simulink model "thermal_closed_loop_model"  (R2023a)
settings: Solver=ode23t  StartTime=0.0  StopTime=600  RelTol=1e-3
PostLoadFcn:
  | run('thermal_model_parameters.m')
  | run('thermal_harness_parameters.m')
  | run('thermal_variants_config.m')
values from neighbouring files (symbols this model uses):
  air_cp = 1004    [cathode_subsystem_parameters.m]    (also in thermal_subsystem_parameters.m)
  air_HC_min = 10    [cathode_subsystem_parameters.m]    (also in thermal_subsystem_parameters.m)
  air_HC_nom = 100    [cathode_subsystem_parameters.m]    (also in thermal_subsystem_parameters.m)
  air_rho = 1.2    [cathode_subsystem_parameters.m]    (also in thermal_subsystem_parameters.m)
  air_vel_nom = 1    [cathode_subsystem_parameters.m]    (also in thermal_subsystem_parameters.m)
  coolant_initial_pressure = 0.111325    [cathode_subsystem_parameters.m]    (also in thermal_subsystem_parameters.m)
  coolant_initial_temperature = 293.15    [cathode_subsystem_parameters.m]    (also in thermal_subsystem_parameters.m)
  coolant_tube_D = 0.05    [cathode_subsystem_parameters.m]    (also in thermal_subsystem_parameters.m)
  Hydrowell_VTS =     [Hydrowell_values_VLV.mat]
  radiator_area_air = 0.10260000000000001    (= 0.1026)    [cathode_subsystem_parameters.m]    (also in thermal_subsystem_parameters.m)
  radiator_area_fins = 2.5436250000000005    (= 2.543625)    [cathode_subsystem_parameters.m]    (also in thermal_subsystem_parameters.m)
  radiator_area_primary = 0.44452500000000011    (= 0.444525)    [cathode_subsystem_parameters.m]    (also in thermal_subsystem_parameters.m = 2 * radiator_tube_length * radiator_width * (radiator_fin_ro)
  radiator_n_tubes = 20    [cathode_subsystem_parameters.m]    (also in thermal_subsystem_parameters.m)
  radiator_tube_height = 0.0015    [cathode_subsystem_parameters.m]    (also in thermal_subsystem_parameters.m)
  radiator_tube_length = 0.45    [cathode_subsystem_parameters.m]    (also in thermal_subsystem_parameters.m)
  radiator_width = 0.025    [cathode_subsystem_parameters.m]    (also in thermal_subsystem_parameters.m)
  tcp_time_constant = 2    [cathode_subsystem_parameters.m]    (also in thermal_subsystem_parameters.m)
undefined symbols (not defined in the file or in its folder): sigbuilder_block, stack
libraries: fl_lib x153, nesl_utility x122, SimscapeFluids_lib x16, slpidlib x5, simulink x1
(part 1 of 8)
settings Model: Creator=adrian.taveras  LastModifiedBy=adrian.taveras
settings SolverCC: MaxConsecutiveMinStep=10
settings OptimizationCC: ReuseModelBlockBuffer=off
settings SimscapeCC: SimscapeLogType=all

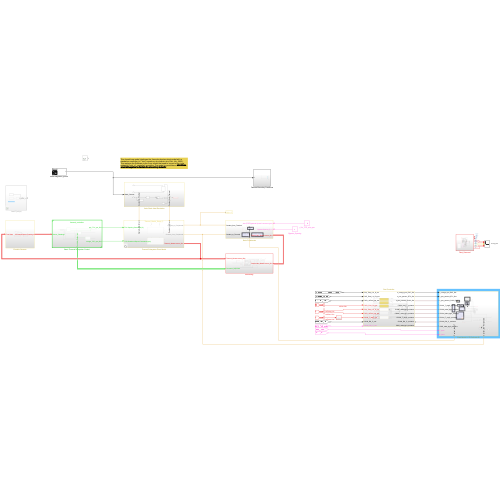
[thumbnail: Simulink's stored preview of the top-level diagram]
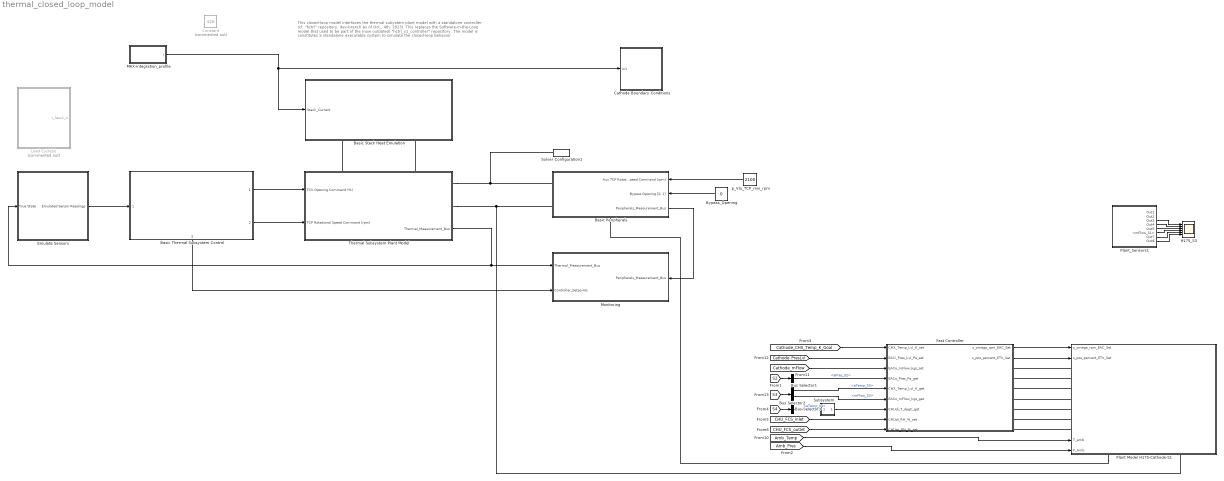
== system thermal_closed_loop_model ==
  note: This closed-loop model interfaces the thermal subystem plant model with a standalone controller (cf. "hctrl" repository, dev-branch as of Oct., 4th, 2023).
      | This replaces the Software-in-the-Loop model that used to be part of the (now outdated) "hctrl_v1_controller" repository. The model is constitutes a standalone executable system to simulate the closed-loop behavior .
  Basic Peripherals : Subsystem
      settings: PortSchema="{\"entries\":[{\"content\":{\"sides\":[{\"content\":{\"connectorIds\":[\"LConn1\",\"LConn2\"]},\"type\":\"ConnectorPlacement.EquallySpacedRectSide\",\"uuid\":\"3fb1bffc-06de-43a0-ba54-014616fc6cc1\"},{\"content\":{\"connectorIds\":[\"In1\",\"In2\",\"Out1\"],\"side\":\"RIGHT\"},\"type\":\"ConnectorPlacement.EquallySpacedRectSide\",\"uuid\":\"58405954-0a26-4c47-92cd-2c539f5c2dc2\"},{\"content\":{\"side\":\"TOP\"},\"type\":\"ConnectorPlacement.EquallySpacedRectSide\",\"uuid\":\"fb935e14-bdb8-42f8-ab88-5e819e25323e\"},{\"content\":{\"connectorIds\":[\"RConn1\"],\"side\":\"BOTTOM\"},\"type\":\"ConnectorPlacement.EquallySpacedRectSide\",\"uuid\":\"4a5f4864-27a3-41f8-b148-25be1e393b46\"}]},\"type\":\"ConnectorPlacement.EquallySpacedConnector\",\"uuid\":\"bd863423-caf1-4028-a014-0e522635d1ca\"}],\"packageUris\":[\"http://schema.mathworks.com/mf0/Connector/R2020b\"],\"version\":\"1.0\"}"
  Basic Stack Heat Emulation : Subsystem
      settings: PortSchema="{\"entries\":[{\"content\":{\"sides\":[{\"content\":{\"connectorIds\":[\"In1\"]},\"type\":\"ConnectorPlacement.EquallySpacedRectSide\",\"uuid\":\"3fb1bffc-06de-43a0-ba54-014616fc6cc1\"},{\"content\":{\"side\":\"RIGHT\"},\"type\":\"ConnectorPlacement.EquallySpacedRectSide\",\"uuid\":\"58405954-0a26-4c47-92cd-2c539f5c2dc2\"},{\"content\":{\"side\":\"TOP\"},\"type\":\"ConnectorPlacement.EquallySpacedRectSide\",\"uuid\":\"fb935e14-bdb8-42f8-ab88-5e819e25323e\"},{\"content\":{\"connectorIds\":[\"RConn1\",\"RConn2\"],\"side\":\"BOTTOM\"},\"type\":\"ConnectorPlacement.EquallySpacedRectSide\",\"uuid\":\"52bc4db1-df79-4132-9e52-2843fbef2d40\"}]},\"type\":\"ConnectorPlacement.EquallySpacedConnector\",\"uuid\":\"bd863423-caf1-4028-a014-0e522635d1ca\"}],\"packageUris\":[\"http://schema.mathworks.com/mf0/Connector/R2020b\"],\"version\":\"1.0\"}"
  Basic Thermal Subsystem Control : Subsystem  TreatAsAtomicUnit=on  SystemSampleTime=0.05  ReferencedSubsystem=thermal_controller
      settings: RTWFcnNameOpts=Use subsystem name  RTWFileNameOpts=Use subsystem name  PortSchema="{\"entries\":[{\"content\":{\"sides\":[{\"content\":{\"connectorIds\":[\"In1\"]},\"type\":\"ConnectorPlacement.EquallySpacedRectSide\",\"uuid\":\"5ce399fd-075d-47cf-80d1-ee07a0b07c67\"},{\"content\":{\"connectorIds\":[\"Out1\",\"Out2\"],\"side\":\"RIGHT\"},\"type\":\"ConnectorPlacement.EquallySpacedRectSide\",\"uuid\":\"2f333d4b-83ed-4fad-b30d-41906106278f\"},{\"content\":{\"side\":\"TOP\"},\"type\":\"ConnectorPlacement.EquallySpacedRectSide\",\"uuid\":\"ce20a072-8b2c-48f8-86cd-e043d93c9dd9\"},{\"content\":{\"connectorIds\":[\"Out3\"],\"side\":\"BOTTOM\"},\"type\":\"ConnectorPlacement.EquallySpacedRectSide\",\"uuid\":\"72f45d63-3937-4d85-84da-630e4ae9e6af\"}]},\"type\":\"ConnectorPlacement.EquallySpacedConnector\",\"uuid\":\"e1990042-c5e7-41f2-bf10-f2665fc49181\"}],\"packageUris\":[\"http://schema.mathworks.com/mf0/Connector/R2020b\"],\"version\":\"1.0\"}"
  Bus Selector1 : BusSelector  OutputSignals=aPres_S2
  Bus Selector2 : BusSelector  OutputSignals=aTemp_S3,mFlow_S3
  Bus Selector3 : BusSelector  OutputSignals=aTemp_S4
  Bypass_Opening : Constant  Value=0
  Cathode Boundary Conditions : Subsystem
  Constant : Constant  Commented=on  Value=426
  Emulate Sensors : Subsystem
  Fast Controller : Subsystem
      settings: PortSchema="{\"entries\":[{\"content\":{\"sides\":[{\"content\":{\"connectorIds\":[\"Out1\",\"Out2\",\"LConn1\",\"LConn2\",\"LConn3\",\"LConn4\",\"LConn5\",\"LConn6\",\"LConn7\"]},\"type\":\"ConnectorPlacement.EquallySpacedRectSide\",\"uuid\":\"fec6d33c-3ad3-4174-acdc-3a3b9e5715f4\"},{\"content\":{\"connectorIds\":[\"In1\",\"In2\",\"In3\",\"In4\",\"In5\",\"In6\",\"In7\",\"In8\",\"In9\"],\"side\":\"RIGHT\"},\"type\":\"ConnectorPlacement.EquallySpacedRectSide\",\"uuid\":\"4aee90de-c0ab-447d-83f7-53a254285efe\"},{\"content\":{\"side\":\"TOP\"},\"type\":\"ConnectorPlacement.EquallySpacedRectSide\",\"uuid\":\"94b2adb1-5e3a-4413-84ea-fe1e13b8a59d\"}]},\"type\":\"ConnectorPlacement.EquallySpacedConnector\",\"uuid\":\"aca8449a-2e64-4d0b-80a0-10fe30b1ea20\"}],\"packageUris\":[\"http://schema.mathworks.com/mf0/Connector/R2020b\"],\"version\":\"1.0\"}"
  H175_S3 : Scope  NumInputPorts=6
  Load Cycle(s) : Subsystem  Commented=on
  MAX-integration_profile : Subsystem  Tag=STV Subsys  LoadFcn=sigbuilder_block('load');  StartFcn=sigbuilder_block('start');  StopFcn=sigbuilder_block('stop');  ClipboardFcn=sigbuilder_block('clipboard');  mask(Sigbuilder block){tuvar=[0:10]}
      mask help: Simulink:masks:SigbuilderBlock_MD
      mask init:
      | if ~strcmp(get_param(bdroot(gcbh),'SimulationStatus'),'stopped') tuvar = sigbuilder_block('maskInit'); end
      settings: CopyFcn=sigbuilder_block('copy');  DeleteFcn=sigbuilder_block('delete');  ModelCloseFcn=sigbuilder_block('modelClose');  PreSaveFcn=sigbuilder_block('preSave');  PauseFcn=sigbuilder_block('pause');  ContinueFcn=sigbuilder_block('continue');  NameChangeFcn=sigbuilder_block('namechange');  OpenFcn=sigbuilder_block('open',[6 30.75 1428 715.5 ]);  CloseFcn=sigbuilder_block('close');
      mask Display: plot(0, 0, 100, 100,[2, 2, 32, 32, 2], [68, 8, 8, 68, 68],[32, 2], [38, 38], [32, 19, 2],[53, 60, 44], [32, 17, 17, 2],[16, 16, 31, 31]);txt = getActiveGroup(gcbh);text(2, 100, txt,'verticalAlignment', 'top');
  Monitoring : Subsystem
      settings: PortSchema="{\"entries\":[{\"content\":{\"sides\":[{\"content\":{\"connectorIds\":[\"In1\",\"In2\"]},\"type\":\"ConnectorPlacement.EquallySpacedRectSide\",\"uuid\":\"c7cb1208-b668-4b39-b890-dd3e20c5f08d\"},{\"content\":{\"connectorIds\":[\"In3\"],\"side\":\"RIGHT\"},\"type\":\"ConnectorPlacement.EquallySpacedRectSide\",\"uuid\":\"340204d2-358d-42ec-bbb6-f536bf598eab\"},{\"content\":{\"side\":\"TOP\"},\"type\":\"ConnectorPlacement.EquallySpacedRectSide\",\"uuid\":\"3db79fdc-6863-4ab5-88bc-fd1ec2b642bb\"}]},\"type\":\"ConnectorPlacement.EquallySpacedConnector\",\"uuid\":\"cd44049f-98c6-404f-bd6e-056e1be05d3b\"}],\"packageUris\":[\"http://schema.mathworks.com/mf0/Connector/R2020b\"],\"version\":\"1.0\"}"
  Plant Model H175-Cathode-S1 : Subsystem
      settings: PortSchema="{\"entries\":[{\"content\":{\"sides\":[{\"content\":{\"connectorIds\":[\"In1\",\"In2\",\"LConn1\",\"LConn2\",\"LConn3\",\"LConn4\",\"LConn5\",\"LConn6\",\"LConn7\",\"In3\",\"In4\"]},\"type\":\"ConnectorPlacement.EquallySpacedRectSide\",\"uuid\":\"e3b30cb5-20d3-4977-927f-9fea068a9234\"},{\"content\":{\"side\":\"RIGHT\"},\"type\":\"ConnectorPlacement.EquallySpacedRectSide\",\"uuid\":\"2d547627-9665-492a-afa4-fcc16b1173a1\"},{\"content\":{\"side\":\"TOP\"},\"type\":\"ConnectorPlacement.EquallySpacedRectSide\",\"uuid\":\"4ee6a80a-af1f-40b1-aa59-916ec7fe1294\"},{\"content\":{\"connectorIds\":[\"RConn1\",\"RConn2\"],\"side\":\"BOTTOM\"},\"type\":\"ConnectorPlacement.EquallySpacedRectSide\",\"uuid\":\"f96b90ea-bf7b-40d9-b9ad-d818d5da9577\"}]},\"type\":\"ConnectorPlacement.EquallySpacedConnector\",\"uuid\":\"0d82e4d1-cc18-4647-90fc-0df577891cdc\"}],\"packageUris\":[\"http://schema.mathworks.com/mf0/Connector/R2020b\"],\"version\":\"1.0\"}"
  Plant_Sensors1 : Subsystem
  Solver Configuration1 : nesl_utility/Solver Configuration  PhysicalDomain=network_engine_domain  SubClassName=solver  LeftPortType=input  RightPortType=generic  Tones=[]  Harmonics=[]  SimulateNoise=off  Profile=off  UseLocalSampling=off  EnableSwitchedLinearOptims=on  FrequencyDomain=off  UseCCode=off  RelTol=0.001  AbsTol=1e-06  MinStep=1e-09  ToWorkspace=off  RevertToSquareIcSolve=off  NumHomotopyIterations=100  PhasorMode=off  PhasorModeNumHarmonics=1  ConsistencySolver=NEWTON_XTOL_AFTER_FTOL  IndexReductionMethod=DerivativeReplacement  DoDC=on  ResidualTolerance=1e-09  ConsistencyTolSource=GLOBAL  ConsistencyAbsTol=0.001  ConsistencyRelTol=0.001  ConsistencyTolFactor=0.001  UseLocalSolver=on  LocalSolverChoice=NE_BACKWARD_EULER_ADVANCER  ResolveIndetEquations=on  FunctionEvalNumThread=1  LocalSolverSampleTime=0.001  DoFixedCost=on  MaxNonlinIter=3  MaxModeIter=2  ComputeImpulses=off  ImpulseIterations=2  LinearAlgebra=auto  LinearAlgebraNumThread=0  EquationFormulation=NE_TIME_EF  DelaysMemoryBudget=1024  AutomaticFiltering=off  FilteringTimeConstant=0.001  PartitionStorageMethod=AS_NEEDED  PartitionMemoryBudget=1024  PartitionMethod=ROBUST
  Subsystem : Subsystem
  Thermal Subsystem Plant Model : Subsystem  Variant=on
      settings: PortSchema="{\"entries\":[{\"content\":{\"sides\":[{\"content\":{\"connectorIds\":[\"In1\",\"In2\"]},\"type\":\"ConnectorPlacement.EquallySpacedRectSide\",\"uuid\":\"c406812b-8c92-4602-a172-62ad771a81a9\"},{\"content\":{\"connectorIds\":[\"RConn1\",\"RConn2\",\"Out1\"],\"side\":\"RIGHT\"},\"type\":\"ConnectorPlacement.EquallySpacedRectSide\",\"uuid\":\"78b6fff5-4256-4005-adaa-354cc2ed5b7d\"},{\"content\":{\"connectorIds\":[\"LConn1\",\"LConn2\"],\"side\":\"TOP\"},\"type\":\"ConnectorPlacement.EquallySpacedRectSide\",\"uuid\":\"1d5f4f72-4393-4f38-b9ce-f5bde53d6a3a\"}]},\"type\":\"ConnectorPlacement.EquallySpacedConnector\",\"uuid\":\"f62a8404-8485-4e42-883e-e8d18b630e2d\"}],\"packageUris\":[\"http://schema.mathworks.com/mf0/Connector/R2020b\"],\"version\":\"1.0\"}"
  p_Vlo_TCP_min_rpm : Constant  Value=2100
  wires:
  Thermal Subsystem Plant Model/1(Thermal_Measurement_Bus) -> Emulate Sensors/1(True State), Monitoring/1(Thermal_Measurement_Bus)
  Emulate Sensors/1(Emulated Sensor Readings) -> Basic Thermal Subsystem Control/1
  p_Vlo_TCP_min_rpm/1 -> Basic Peripherals/1(Aux TCP Rotational Speed Command (rpm))
  Basic Peripherals/1(Peripherals_Measurement_Bus) -> Monitoring/3(Peripherals_Measurement_Bus)
  Basic Thermal Subsystem Control/3 -> Monitoring/2(Controller_Setpoints)
  Bypass_Opening/1 -> Basic Peripherals/2("Bypass Opening [0, 1]")
  Basic Thermal Subsystem Control/1 -> Thermal Subsystem Plant Model/1(TCV Opening Command (%))
  Basic Thermal Subsystem Control/2 -> Thermal Subsystem Plant Model/2(TCP Rotational Speed Command (rpm))
  [Amb_Temp] -> Plant Model H175-Cathode-S1/3(T_amb)
  Bus Selector1/1 -> Fast Controller/4(EACo_Pres_Pa_get)  "<aPres_S2>"
  Bus Selector3/1 -> Subsystem/1(<aTemp_S4>)  "<aTemp_S4>"
  Bus Selector2/1 -> Fast Controller/5(CHX_Temp_Lvl_K_get)  "<aTemp_S3>"
  [S3] -> Bus Selector2/1
  [Cathode_CHX_Temp_K_Goal] -> Fast Controller/1(CHX_Temp_Lvl_K_set)
  Fast Controller/2(s_pos_percent_ETV_Set) -> Plant Model H175-Cathode-S1/2(s_pos_percent_ETV_Set)
  Fast Controller/1(s_omega_rpm_EAC_Set) -> Plant Model H175-Cathode-S1/1(s_omega_rpm_EAC_Set)
  [CHU_FCS_outlet] -> Fast Controller/9(CHUwi_RH_%_set)
  Bus Selector2/2 -> Fast Controller/6(EACo_mFlow_kgs_get)  "<mFlow_S3>"
  Subsystem/1(Out1) -> Fast Controller/7(CHUdi_T_degC_get)
  [S4] -> Bus Selector3/1
  Plant_Sensors1/7(Out7) -> H175_S3/5
  [Cathode_PresLvl] -> Fast Controller/2(EACi_Pres_Lvl_Pa_set)
  [CHU_FCS_inlet] -> Fast Controller/8(CHUdi_RH_%_set)
  Plant_Sensors1/5(Out5) -> H175_S3/3
  Plant_Sensors1/4(Out4) -> H175_S3/2
  Plant_Sensors1/3(Out3) -> H175_S3/1
  Plant_Sensors1/8(Out8) -> H175_S3/6
  [Cathode_mFlow] -> Fast Controller/3(EACo_mFlow_kgs_set)
  [S2] -> Bus Selector1/1
  MAX-integration_profile/1(I) -> Basic Stack Heat Emulation/1(Stack_Current), Cathode Boundary Conditions/1(In1)
  Plant_Sensors1/6(<mFlow_S1>) -> H175_S3/4
  [Amb_Pres] -> Plant Model H175-Cathode-S1/4(P_Amb)
  connections:
  Thermal Subsystem Plant Model/LConn2 -- Basic Stack Heat Emulation/RConn2
  Thermal Subsystem Plant Model/LConn1 -- Basic Stack Heat Emulation/RConn1
  Solver Configuration1/RConn1 -- Thermal Subsystem Plant Model/RConn1 -- Basic Peripherals/LConn1
  Thermal Subsystem Plant Model/RConn2 -- Plant Model H175-Cathode-S1/RConn2 -- Basic Peripherals/LConn2
  Plant Model H175-Cathode-S1/LConn6 -- Fast Controller/LConn6
  Plant Model H175-Cathode-S1/LConn7 -- Fast Controller/LConn7
  Plant Model H175-Cathode-S1/LConn4 -- Fast Controller/LConn4
  Plant Model H175-Cathode-S1/LConn5 -- Fast Controller/LConn5
  Plant Model H175-Cathode-S1/LConn2 -- Fast Controller/LConn2
  Plant Model H175-Cathode-S1/LConn3 -- Fast Controller/LConn3
  Plant Model H175-Cathode-S1/LConn1 -- Fast Controller/LConn1
  Plant Model H175-Cathode-S1/RConn1 -- Basic Peripherals/RConn1

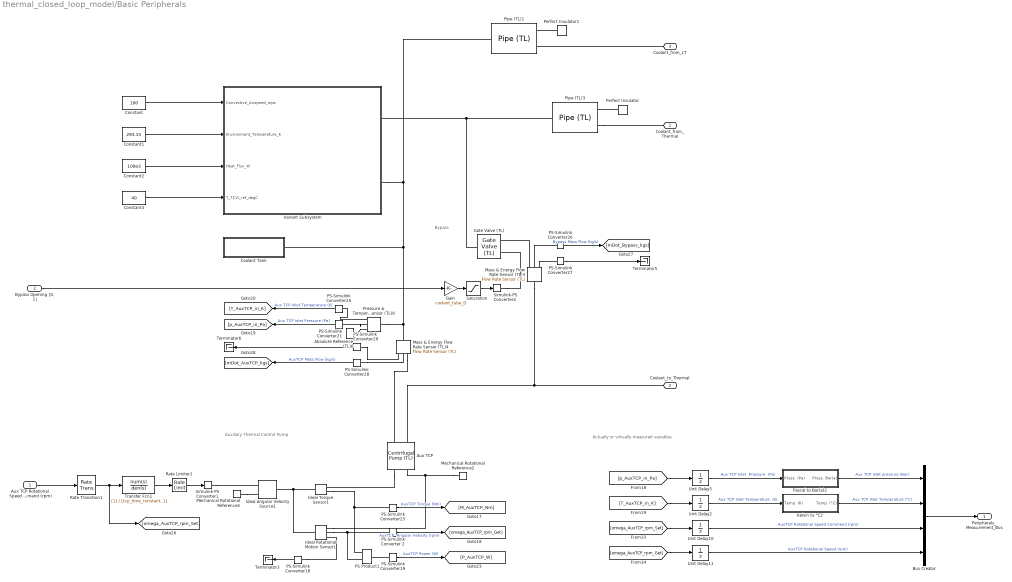
== system thermal_closed_loop_model/Basic Peripherals ==
  note: Auxiliary Thermal Control Pump
  note: Actually or virtually measured variables
  note: Bypass
  Aux TCP Rotational Speed Command (rpm) : Inport
  "Bypass Opening [0, 1]" : Inport  Port=2
  Absolute Reference (TL)6 : fl_lib/Thermal Liquid/Elements/Absolute Reference (TL)
  Aux TCP : SimscapeFluids_lib/Thermal Liquid/Pumps & Motors/Centrifugal Pump (TL)  pump_parameterization=fluids.thermal_liquid.pumps_motors.enum.CentrifugalPumpParameterization.Nominal  capacity_ref_nominal=6000/60 lpm  head_ref_nominal=|  power_ref_nominal=0.3 kW  head_ref_max=|  capacity_ref_max=12000/60 lpm  omega_ref_analytic=3500 rpm  flow_rate_1D_TLU=[1000, 2000, 3000, 4000, 5000, 6000, 7000, 8000, 9000, 1000] lpm  head_1D_TLU=[50, 47.5, 45, 40, 35, 25] m  power_1D_TLU=[.6, .75, .85, .93, .98, .99] kW  omega_ref_1D=3500 rpm  rho_ref_1D=998.21 kg/m^3  omega_threshold_factor=1e-2  flow_rate_2D_TLU=[16.67, 23.33, 30, 40, 53.33, 60] lpm  omega_2D_TLU=[2450, 2800, 3150, 3500] rpm  head_2D_TLU=[25, 32.7, 42.5, 50; 24, 31.7, 41, 49; 22.7, 30.5, 39, 47.5; 20, 28, 36, 45; 15.7, 24, 32, 40; 12.5, 21, 29.5, 37.5] m  power_2D_TLU=[.28, .38, .5, .6; .31, .41, .55, .68; .33, .44, .6, .75; .36, .48, .65, .83; .38, .53, .72, .93; .39, .55, .75, .97] kW  rho_ref_2D=998.21 kg/m^3  diameter_ratio=1  mech_orientation=fluids.thermal_liquid.pumps_motors.enum.CentrifugalPumpMechOrientation.Positive  area=9.6211275016187417927918453612935e-4 m^2
      head_ref_nominal=|
      | 1.2*10^5/(1000*9.81)
      |  m
      head_ref_max=|
      | 1.55*10^5/(1000*9.81)
      |  m
      settings: InternalSimscapePortConfiguration="{\"Bottom\":[],\"Left\":[{\"id\":\"A\",\"label\":\"A\",\"type\":\"foundation.thermal_liquid.thermal_liquid\"},{\"id\":\"B\",\"label\":\"B\",\"type\":\"foundation.thermal_liquid.thermal_liquid\"}],\"Right\":[{\"id\":\"R\",\"label\":\"R\",\"type\":\"foundation.mechanical.rotational.rotational\"},{\"id\":\"C\",\"label\":\"C\",\"type\":\"foundation.mechanical.rotational.rotational\"}],\"Top\":[]}"
  Bus Creator : BusCreator  Inputs=4
  Constant : Constant  Value=100
  Constant1 : Constant  Value=293.15
  Constant2 : Constant  Value=100e3
  Constant3 : Constant  Value=40
  Coolant Tank : Subsystem  Tag=PublishSubsystem  mask(Coolant Tank){A=1, x_init=0.08}
      mask prompts: A "Tank area (m^2)"; x_init "Initial coolant level (m)"
      mask help: This subsystem models an expansion tank for the coolant system.
  Gain : Gain  Gain=coolant_tube_D
  Gate Valve (TL) : SimscapeFluids_lib/Thermal Liquid/Valves & Orifices/Flow Control Valves/Gate Valve (TL)  diam_orifice=coolant_tube_D*0.9 m  S_min=0 m  area_leak=1e-12 m^2  smoothing_factor=0.01  area=pi*coolant_tube_D^2/4 m^2  Cd=0.7  Re_c=12
      settings: InternalSimscapePortConfiguration="{\"Bottom\":[],\"Left\":[{\"id\":\"A\",\"label\":\"A\",\"type\":\"foundation.thermal_liquid.thermal_liquid\"},{\"id\":\"S\",\"label\":\"S\",\"type\":\"input\"}],\"Right\":[{\"id\":\"B\",\"label\":\"B\",\"type\":\"foundation.thermal_liquid.thermal_liquid\"}],\"Top\":[]}"
  Ideal Angular Velocity Source1 : fl_lib/Mechanical/Mechanical Sources/Ideal Angular Velocity Source
  Ideal Rotational Motion Sensor1 : fl_lib/Mechanical/Mechanical Sensors/Ideal Rotational Motion Sensor  reference=foundation.enum.MeasurementReference.difference  acceleration_port=false  velocity_port=true  position_port=true  wrap_angle=false  offset=0 rad
  Ideal Torque Sensor1 : fl_lib/Mechanical/Mechanical Sensors/Ideal Torque Sensor
  Kelvin to °C2 : Subsystem
  Mass & Energy Flow Rate Sensor (TL)3 : fl_lib/Thermal Liquid/Sensors/Flow Rate Sensor (TL)  mass_flow_measure=true  volumetric_flow_measure=false  energy_flow_measure=true
      settings: InternalSimscapePortConfiguration="{\"Bottom\":[{\"id\":\"PHI\",\"label\":\"φ\",\"type\":\"output\"}],\"Left\":[{\"id\":\"A\",\"label\":\"A\",\"type\":\"foundation.thermal_liquid.thermal_liquid\"}],\"Right\":[{\"id\":\"B\",\"label\":\"B\",\"type\":\"foundation.thermal_liquid.thermal_liquid\"},{\"id\":\"M\",\"label\":\"M\",\"type\":\"output\"}],\"Top\":[]}"
  Mass & Energy Flow Rate Sensor (TL)4 : fl_lib/Thermal Liquid/Sensors/Flow Rate Sensor (TL)  mass_flow_measure=true  volumetric_flow_measure=false  energy_flow_measure=true
      settings: InternalSimscapePortConfiguration="{\"Bottom\":[{\"id\":\"PHI\",\"label\":\"φ\",\"type\":\"output\"}],\"Left\":[{\"id\":\"A\",\"label\":\"A\",\"type\":\"foundation.thermal_liquid.thermal_liquid\"}],\"Right\":[{\"id\":\"B\",\"label\":\"B\",\"type\":\"foundation.thermal_liquid.thermal_liquid\"},{\"id\":\"M\",\"label\":\"M\",\"type\":\"output\"}],\"Top\":[]}"
  Mechanical Rotational Reference2 : fl_lib/Mechanical/Rotational Elements/Mechanical Rotational Reference
  Mechanical Rotational Reference4 : fl_lib/Mechanical/Rotational Elements/Mechanical Rotational Reference
  PS Product1 : fl_lib/Physical Signals/Functions/PS Product
  PS-Simulink Converter 2 : nesl_utility/PS-Simulink Converter  PhysicalDomain=network_engine_domain  SubClassName=ps_output  LeftPortType=input  RightPortType=output  PseudoPeriodic=off  Frequencies=[]  VectorFormat=1-D array  Unit=rpm  AffineConversion=off
  PS-Simulink Converter{18,20..21,26..29} (7 alike) : nesl_utility/PS-Simulink Converter  PhysicalDomain=network_engine_domain  SubClassName=ps_output  LeftPortType=input  RightPortType=output  PseudoPeriodic=off  Frequencies=[]  VectorFormat=inherit  Unit=inherit  AffineConversion=off
  PS-Simulink Converter19 : nesl_utility/PS-Simulink Converter  PhysicalDomain=network_engine_domain  SubClassName=ps_output  LeftPortType=input  RightPortType=output  PseudoPeriodic=off  Frequencies=[]  VectorFormat=inherit  Unit=W  AffineConversion=off
  PS-Simulink Converter25 : nesl_utility/PS-Simulink Converter  PhysicalDomain=network_engine_domain  SubClassName=ps_output  LeftPortType=input  RightPortType=output  PseudoPeriodic=off  Frequencies=[]  VectorFormat=inherit  Unit=N*m  AffineConversion=off
  Pascal to Bar(a)2 : Subsystem
  Perfect Insulator : fl_lib/Thermal/Thermal Elements/Perfect Insulator  T_specify=off  T_priority=None  T=293.15 K  T_nominal_specify=off  T_nominal_unit=K  T_nominal_value=1
  Perfect Insulator1 : fl_lib/Thermal/Thermal Elements/Perfect Insulator  T_specify=off  T_priority=None  T=293.15 K  T_nominal_specify=off  T_nominal_unit=K  T_nominal_value=1
  Pipe (TL)1 : fl_lib/Thermal Liquid/Elements/Pipe (TL)  length=1 m  area=pi*(coolant_tube_D/2)^2/4 m^2  Dh=pi*coolant_tube_D*.5*0.9 m  length_add=1 m  roughness=15e-6 m  Re_lam=2000  Re_tur=4000  shape_factor=64  Nu_lam=3.66  dynamic_compressibility=simscape.enum.onoff.on  inertia=simscape.enum.onoff.off  p0=coolant_initial_pressure MPa  T0=coolant_initial_temperature K  mdot0=0 kg/s
  Pipe (TL)3 : fl_lib/Thermal Liquid/Elements/Pipe (TL)  length=1 m  area=pi*coolant_tube_D^2/4 m^2  Dh=pi*coolant_tube_D*0.9 m  length_add=1 m  roughness=15e-6 m  Re_lam=2000  Re_tur=4000  shape_factor=64  Nu_lam=3.66  dynamic_compressibility=simscape.enum.onoff.on  inertia=simscape.enum.onoff.off  p0=coolant_initial_pressure MPa  T0=coolant_initial_temperature K  mdot0=0 kg/s
  Pressure & Temperature Sensor (TL)6 : fl_lib/Thermal Liquid/Sensors/Pressure & Temperature Sensor (TL)  reference=foundation.enum.MeasurementReference.difference  pressure=true  pressure_spec=foundation.enum.PressureMeasementSpec.Absolute  temperature=true
      settings: InternalSimscapePortConfiguration="{\"Bottom\":[{\"id\":\"T\",\"label\":\"T\",\"type\":\"output\"}],\"Left\":[{\"id\":\"A\",\"label\":\"A\",\"type\":\"foundation.thermal_liquid.thermal_liquid\"}],\"Right\":[{\"id\":\"B\",\"label\":\"B\",\"type\":\"foundation.thermal_liquid.thermal_liquid\"},{\"id\":\"P\",\"label\":\"P\",\"type\":\"output\"}],\"Top\":[]}"
  Rate Limiter1 : RateLimiter  RisingSlewLimit=1000  FallingSlewLimit=-1000  SampleTimeMode=inherited
  Rate Transition1 : RateTransition
  Saturation : Saturate  UpperLimit=coolant_tube_D  LowerLimit=0
  Simulink-PS Converter1 : nesl_utility/Simulink-PS Converter  PhysicalDomain=network_engine_domain  SubClassName=ps_input  LeftPortType=input  RightPortType=output  PseudoPeriodic=off  Frequencies=[]  NoiseDistribution=none  NoiseParameters=[]  Unit=rpm  AffineConversion=off  FilteringAndDerivatives=provide  SimscapeFilterOrder=1  InputFilterTimeConstant=0.001  UdotUserProvided=0
  Simulink-PS Converter4 : nesl_utility/Simulink-PS Converter  PhysicalDomain=network_engine_domain  SubClassName=ps_input  LeftPortType=input  RightPortType=output  PseudoPeriodic=off  Frequencies=[]  NoiseDistribution=none  NoiseParameters=[]  Unit=1  AffineConversion=off  FilteringAndDerivatives=provide  SimscapeFilterOrder=1  InputFilterTimeConstant=0.001  UdotUserProvided=0
  Terminator3 : Terminator
  Terminator5 : Terminator
  Terminator6 : Terminator
  Transfer Fcn1 : TransferFcn  Denominator=[tcp_time_constant, 1]  ContinuousStateAttributes='tcv_opening'
  Unit Delay10 : UnitDelay  SampleTime=-1  HasFrameUpgradeWarning=on
  Unit Delay11 : UnitDelay  SampleTime=-1  HasFrameUpgradeWarning=on
  Unit Delay2 : UnitDelay  InitialCondition=coolant_initial_temperature  SampleTime=-1  HasFrameUpgradeWarning=on
  Unit Delay5 : UnitDelay  InitialCondition=coolant_initial_pressure  SampleTime=-1  HasFrameUpgradeWarning=on
  Variant Subsystem : Subsystem  Variant=on
  Coolant_from_Thermal : PMIOPort  Side=Left
  Coolant_to_Thermal : PMIOPort  Port=2  Side=Left
  Coolant_from_LT : PMIOPort  Port=3  Side=Right
  Peripherals_Measurement_Bus : Outport
  wires:
  Aux TCP Rotational Speed Command (rpm)/1 -> Rate Transition1/1
  PS-Simulink Converter29/1 -> Terminator6/1
  PS-Simulink Converter20/1 -> [T_AuxTCP_in_K]  "Aux TCP Inlet Temperature (K)"
  PS-Simulink Converter21/1 -> [p_AuxTCP_in_Pa]  "Aux TCP Inlet Pressure (Pa)"
  PS-Simulink Converter19/1 -> [P_AuxTCP_W]  "AuxTCP Power (W)"
  Rate Transition1/1 -> [omega_AuxTCP_rpm_Set], Transfer Fcn1/1
  PS-Simulink Converter 2/1 -> [omega_AuxTCP_rpm_Get]  "AuxTCP  Angular Velocity (rpm)"
  PS-Simulink Converter25/1 -> [M_AuxTCP_Nm]  "AuxTCP Torque (Nm)"
  PS-Simulink Converter18/1 -> Terminator3/1
  Rate Limiter1/1 -> Simulink-PS Converter1/1
  Transfer Fcn1/1 -> Rate Limiter1/1
  PS-Simulink Converter28/1 -> [mDot_AuxTCP_kgs]  "AuxTCP Mass Flow (kg/s)"
  Pascal to Bar(a)2/1(Press. Bar(a)) -> Bus Creator/1  "Aux TCP Inlet pressure (Bar)"
  Unit Delay10/1 -> Bus Creator/3  "AuxTCP Rotational Speed Command (rpm)"
  Kelvin to °C2/1(Temp. (°C)) -> Bus Creator/2  "Aux TCP Inlet Temperature (°C)"
  [omega_AuxTCP_rpm_Get] -> Unit Delay11/1
  Unit Delay2/1 -> Kelvin to °C2/1(Temp. (K))  "Aux TCP Inlet Temperature  (K)"
  Unit Delay5/1 -> Pascal to Bar(a)2/1(Press. (Pa))  "Aux TCP Inlet  Pressure  (Pa)"
  Unit Delay11/1 -> Bus Creator/4  "AuxTCP Rotational Speed (rpm)"
  [p_AuxTCP_in_Pa] -> Unit Delay5/1
  [T_AuxTCP_in_K] -> Unit Delay2/1
  [omega_AuxTCP_rpm_Set] -> Unit Delay10/1
  Bus Creator/1 -> Peripherals_Measurement_Bus/1
  Constant/1 -> Variant Subsystem/1(Convective_Airspeed_mps)
  Constant1/1 -> Variant Subsystem/2(Environment_Temperature_K)
  Constant2/1 -> Variant Subsystem/3(Heat_Flux_W)
  Constant3/1 -> Variant Subsystem/4(T_TCVi_ref_degC)
  PS-Simulink Converter26/1 -> [mDot_Bypass_kgs]  "Bypass Mass Flow (kg/s)"
  PS-Simulink Converter27/1 -> Terminator5/1
  Gain/1 -> Saturation/1
  "Bypass Opening [0, 1]"/1 -> Gain/1
  Saturation/1 -> Simulink-PS Converter4/1
  connections:
  Mechanical Rotational Reference2/LConn1 -- Ideal Rotational Motion Sensor1/RConn1 -- Aux TCP/RConn2
  Pressure & Temperature Sensor (TL)6/LConn1 -- Mass & Energy Flow Rate Sensor (TL)4/LConn1 -- Pipe (TL)1/RConn1 -- Variant Subsystem/RConn2 -- Coolant Tank/RConn1
  Ideal Angular Velocity Source1/LConn1 -- Ideal Torque Sensor1/LConn1 -- Ideal Rotational Motion Sensor1/LConn1
  Ideal Rotational Motion Sensor1/RConn2 -- PS-Simulink Converter 2/LConn1 -- PS Product1/LConn2
  Ideal Torque Sensor1/RConn2 -- PS Product1/LConn1 -- PS-Simulink Converter25/LConn1
  Simulink-PS Converter1/RConn1 -- Ideal Angular Velocity Source1/RConn1
  PS-Simulink Converter28/LConn1 -- Mass & Energy Flow Rate Sensor (TL)4/RConn2
  Pressure & Temperature Sensor (TL)6/RConn1 -- Absolute Reference (TL)6/LConn1
  Pressure & Temperature Sensor (TL)6/RConn2 -- PS-Simulink Converter21/LConn1
  Aux TCP/RConn1 -- Ideal Torque Sensor1/RConn1
  Mechanical Rotational Reference4/LConn1 -- Ideal Angular Velocity Source1/RConn2
  PS-Simulink Converter18/LConn1 -- Ideal Rotational Motion Sensor1/RConn3
  PS-Simulink Converter19/LConn1 -- PS Product1/RConn1
  Mass & Energy Flow Rate Sensor (TL)4/RConn1 -- Aux TCP/LConn1
  Pressure & Temperature Sensor (TL)6/RConn3 -- PS-Simulink Converter20/LConn1
  PS-Simulink Converter29/LConn1 -- Mass & Energy Flow Rate Sensor (TL)4/RConn3
  Aux TCP/LConn2 -- Mass & Energy Flow Rate Sensor (TL)3/LConn1 -- Coolant_to_Thermal/RConn1
  Gate Valve (TL)/RConn1 -- Pipe (TL)3/RConn1 -- Variant Subsystem/RConn1
  Mass & Energy Flow Rate Sensor (TL)3/RConn1 -- Gate Valve (TL)/LConn1
  PS-Simulink Converter26/LConn1 -- Mass & Energy Flow Rate Sensor (TL)3/RConn2
  Simulink-PS Converter4/RConn1 -- Gate Valve (TL)/LConn2
  PS-Simulink Converter27/LConn1 -- Mass & Energy Flow Rate Sensor (TL)3/RConn3
  Pipe (TL)3/LConn1 -- Coolant_from_Thermal/RConn1
  Perfect Insulator/LConn1 -- Pipe (TL)3/LConn2
  Perfect Insulator1/LConn1 -- Pipe (TL)1/LConn2
  Coolant_from_LT/RConn1 -- Pipe (TL)1/LConn1

== system thermal_closed_loop_model/Basic Stack Heat Emulation ==
  Stack_Current : Inport
  Controlled Heat Flow Rate Source1 : fl_lib/Thermal/Thermal Sources/Controlled Heat Flow Rate Source
  Current to Heat (W) : Lookup_n-D  NumberOfTableDimensions=1  BreakpointsForDimension1=[0:50:400]  Table=[0, 9932, 21438, 33442,47123, 59491, 77033, 93585, 112042]  InternalRulePriority=Speed  RndMeth=Simplest
  Fuel Cell Coolant Channels : fl_lib/Thermal Liquid/Elements/Pipe (TL)  length=sqrt(stack.area) * stack.coolant_num_passes cm  area=stack.coolant_w_channels^2 * stack.coolant_num_layers cm^2  Dh=stack.coolant_w_channels cm  length_add=10 cm  roughness=15e-5 m  Re_lam=2000  Re_tur=4000  shape_factor=64  Nu_lam=3.66  dynamic_compressibility=simscape.enum.onoff.on  inertia=simscape.enum.onoff.off  p0=coolant_initial_pressure MPa  T0=coolant_initial_temperature K  mdot0=0 kg/s
  Heat Flow Rate Sensor1 : fl_lib/Thermal/Thermal Sensors/Heat Flow Rate Sensor
  PS-Simulink Converter16 : nesl_utility/PS-Simulink Converter  PhysicalDomain=network_engine_domain  SubClassName=ps_output  LeftPortType=input  RightPortType=output  PseudoPeriodic=off  Frequencies=[]  VectorFormat=1-D array  Unit=kW  AffineConversion=off
  PS100-P02Stack Thermal Mass : fl_lib/Thermal/Thermal Elements/Thermal Mass  mass_type=foundation.enum.constant_variable.constant  mass=stack.thermal_mass kg  sp_heat=stack.specific_heat J/kg/K  mass_min=1e-6 kg  num_ports=foundation.enum.numPorts2.one  m_specify=off  m_priority=High  m=1 kg  m_nominal_specify=off  m_nominal_unit=kg  m_nominal_value=1  T_specify=on  T_priority=High  T=coolant_initial_temperature K  T_nominal_specify=off  T_nominal_unit=K  T_nominal_value=1  Q_specify=off  Q_priority=None  Q=20e3 W  Q_nominal_specify=off  Q_nominal_unit=W  Q_nominal_value=1
  Simulink-PS Converter6 : nesl_utility/Simulink-PS Converter  PhysicalDomain=network_engine_domain  SubClassName=ps_input  LeftPortType=input  RightPortType=output  PseudoPeriodic=off  Frequencies=[]  NoiseDistribution=none  NoiseParameters=[]  Unit=J/s  AffineConversion=off  FilteringAndDerivatives=provide  SimscapeFilterOrder=1  InputFilterTimeConstant=0.001  UdotUserProvided=0
  Thermal Reference1 : fl_lib/Thermal/Thermal Elements/Thermal Reference
  Coolant_to_Thermal : PMIOPort  Side=Right
  Coolant_from_Thermal : PMIOPort  Port=2  Side=Right
  tag scope: I_SFC_A=global, Q_Stack_kW=global
  wires:
  Current to Heat (W)/1 -> Simulink-PS Converter6/1
  PS-Simulink Converter16/1 -> [Q_Stack_kW]
  Stack_Current/1 -> Current to Heat (W)/1, [I_SFC_A]
  connections:
  Thermal Reference1/LConn1 -- Controlled Heat Flow Rate Source1/RConn2
  Controlled Heat Flow Rate Source1/LConn1 -- Heat Flow Rate Sensor1/LConn1
  Fuel Cell Coolant Channels/LConn2 -- Heat Flow Rate Sensor1/RConn2 -- PS100-P02Stack Thermal Mass/LConn1
  Heat Flow Rate Sensor1/RConn1 -- PS-Simulink Converter16/LConn1
  Simulink-PS Converter6/RConn1 -- Controlled Heat Flow Rate Source1/RConn1
  Coolant_from_Thermal/RConn1 -- Fuel Cell Coolant Channels/LConn1
  Coolant_to_Thermal/RConn1 -- Fuel Cell Coolant Channels/RConn1

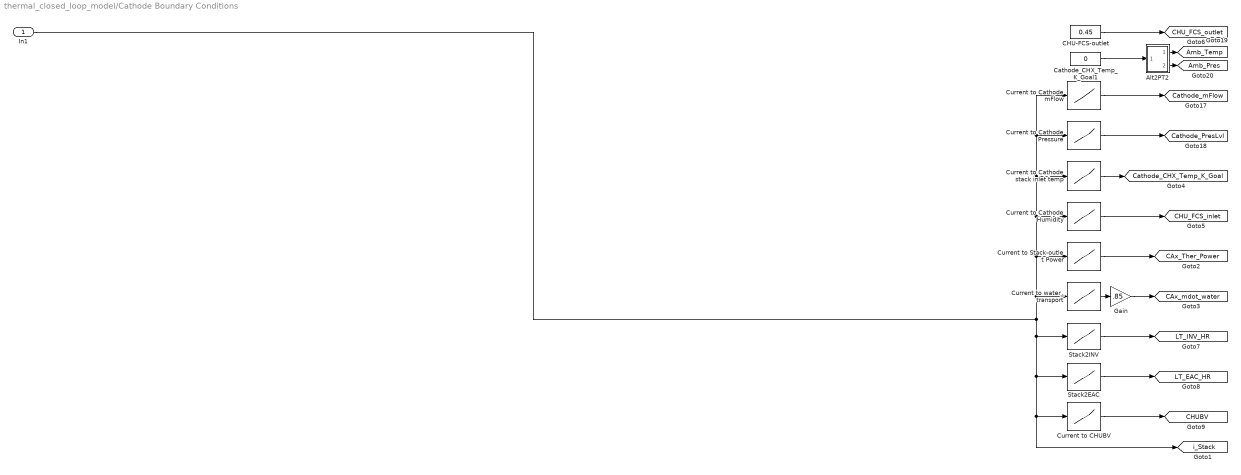
== system thermal_closed_loop_model/Cathode Boundary Conditions ==
  In1 : Inport
  Alt2PT2 : Subsystem
  CHU-FCS-outlet : Constant  Value=0.45
  Cathode_CHX_Temp_K_Goal1 : Constant  Value=0
  Current to CHUBV : Lookup_n-D  NumberOfTableDimensions=1  BreakpointsForDimension1=[0;100;200;350;400;500;600]  Table=[0;0;0;1;1;1;1]  InternalRulePriority=Speed  RndMeth=Simplest
  Current to Cathode Humidity : Lookup_n-D  NumberOfTableDimensions=1  BreakpointsForDimension1=[20, 50, 100, 150, 200, 250, 300, 350, 400, 450, 500, 550, 600]  Table=[0.8,0.77,0.75,0.72,0.7,0.65,0.65,0.6,0.55,0.55,0.53,0.53,0.53]  InternalRulePriority=Speed  RndMeth=Simplest
  Current to Cathode Pressure : Lookup_n-D  NumberOfTableDimensions=1  BreakpointsForDimension1=[0;50;100;150;200;300;400;450;500;550;600]  Table=[112000;112000;170000;175000;180000;210000;210000;210000;210000;210000;230000]  InternalRulePriority=Speed  RndMeth=Simplest
  Current to Cathode mFlow : Lookup_n-D  NumberOfTableDimensions=1  BreakpointsForDimension1=[0;50;100;150;200;250;300;350;400;510;600]  Table=[0;0.03;0.05;0.07;0.0825;0.095;0.095;0.105;0.123;0.152;0.167]  InternalRulePriority=Speed  RndMeth=Simplest
  Current to Cathode stack inlet temp : Lookup_n-D  NumberOfTableDimensions=1  BreakpointsForDimension1=[20, 50, 100, 150, 200, 250, 300, 350, 400, 450, 500, 550, 600]  Table=[65,65,66,67,68,68,68,68,69,70,70,70,70]  InternalRulePriority=Speed  RndMeth=Simplest
  Current to Stack-outlet Power : Lookup_n-D  NumberOfTableDimensions=1  BreakpointsForDimension1=[20, 50, 100, 150, 200, 250, 300, 350, 400, 450, 500, 550, 600]  Table=[0.0274, 0.1198, 0.1925, 0.2134, 0.2502, 0.3358, 0.4478, 0.5224, 0.5988, 0.6756, 0.8257, 0.9909, 1.0339]*1000  InternalRulePriority=Speed  RndMeth=Simplest
  Current to water_transport : Lookup_n-D  NumberOfTableDimensions=1  BreakpointsForDimension1=[0;100;200;400;600]  Table=[0;4.247e-3;8.494e-3;1.697e-2;2.548e-2]  InternalRulePriority=Speed  RndMeth=Simplest
  Gain : Gain  Gain=.85
  Stack2EAC : Lookup_n-D  NumberOfTableDimensions=1  BreakpointsForDimension1=[0 100 200 300 400 500 600]  Table=[0;610;940;1760;3980;4620;5190]  InternalRulePriority=Speed  RndMeth=Simplest
  Stack2INV : Lookup_n-D  NumberOfTableDimensions=1  BreakpointsForDimension1=[0;100;200;300;400;500;600]  Table=[0;550;690;1450;2490;2870;2920]  InternalRulePriority=Speed  RndMeth=Simplest
  tag scope: Amb_Pres=global, Amb_Temp=global, CAx_Ther_Power=global, CAx_mdot_water=global, CHUBV=global, CHU_FCS_inlet=global, CHU_FCS_outlet=global, Cathode_CHX_Temp_K_Goal=global, Cathode_PresLvl=global, Cathode_mFlow=global, LT_EAC_HR=global, LT_INV_HR=global, i_Stack=global
  wires:
  Current to Stack-outlet Power/1 -> [CAx_Ther_Power]
  Current to CHUBV/1 -> [CHUBV]
  Current to Cathode stack inlet temp/1 -> [Cathode_CHX_Temp_K_Goal]
  In1/1 -> Current to Cathode mFlow/1, Current to Cathode Pressure/1, Current to Cathode stack inlet temp/1, Current to Cathode Humidity/1, Current to Stack-outlet Power/1, Current to water_transport/1, Current to CHUBV/1, [i_Stack], Stack2EAC/1, Stack2INV/1
  Current to water_transport/1 -> Gain/1
  Stack2INV/1 -> [LT_INV_HR]
  Stack2EAC/1 -> [LT_EAC_HR]
  Gain/1 -> [CAx_mdot_water]
  Alt2PT2/1(Out1) -> [Amb_Temp]
  Current to Cathode Humidity/1 -> [CHU_FCS_inlet]
  Current to Cathode mFlow/1 -> [Cathode_mFlow]
  CHU-FCS-outlet/1 -> [CHU_FCS_outlet]
  Alt2PT2/2(Out2) -> [Amb_Pres]
  Cathode_CHX_Temp_K_Goal1/1 -> Alt2PT2/1(In1)
  Current to Cathode Pressure/1 -> [Cathode_PresLvl]

== system thermal_closed_loop_model/Emulate Sensors ==
  True State : Inport
  Band-Limited White Noise : simulink/Sources/Band-Limited White Noise  Cov=[5e-3, 5e-4, 5e-4]  Ts=0.1  seed=[23341]
  Bus Creator : BusCreator  Inputs=3
  Bus Selector : BusSelector  OutputSignals=Stack Current: I_A_StN (A),Stack Inlet Temperature: TSens_CLSti 6812 (°C),Stack Outlet Temperature: TSens_CLSto 6820 (°C)
  Constant : Constant  Value=zeros(1,3)
  Demux : Demux  Outputs=3
  Manual Switch : ManualSwitch  CurrentSetting=0
  Mux : Mux  Inputs=3
  Sum : Sum  Inputs=++|
  Emulated Sensor Readings : Outport
  wires:
  Bus Creator/1 -> Emulated Sensor Readings/1
  True State/1 -> Bus Selector/1
  Bus Selector/1 -> Mux/1  "<Stack Current: I_A_StN (A)>"
  Bus Selector/2 -> Mux/2  "<Stack Inlet Temperature: TSens_CLSti 6812 (°C)>"
  Bus Selector/3 -> Mux/3  "<Stack Outlet Temperature: TSens_CLSto 6820 (°C)>"
  Mux/1 -> Sum/2
  Sum/1 -> Demux/1
  Manual Switch/1 -> Sum/1
  Band-Limited White Noise/1 -> Manual Switch/1  "Signal Noise"
  Constant/1 -> Manual Switch/2
  Demux/1 -> Bus Creator/1  "s_I_A_StN_Get"
  Demux/3 -> Bus Creator/3  "s_T_decC_CLSto_Get"
  Demux/2 -> Bus Creator/2  "s_T_decC_CLSti_Get"

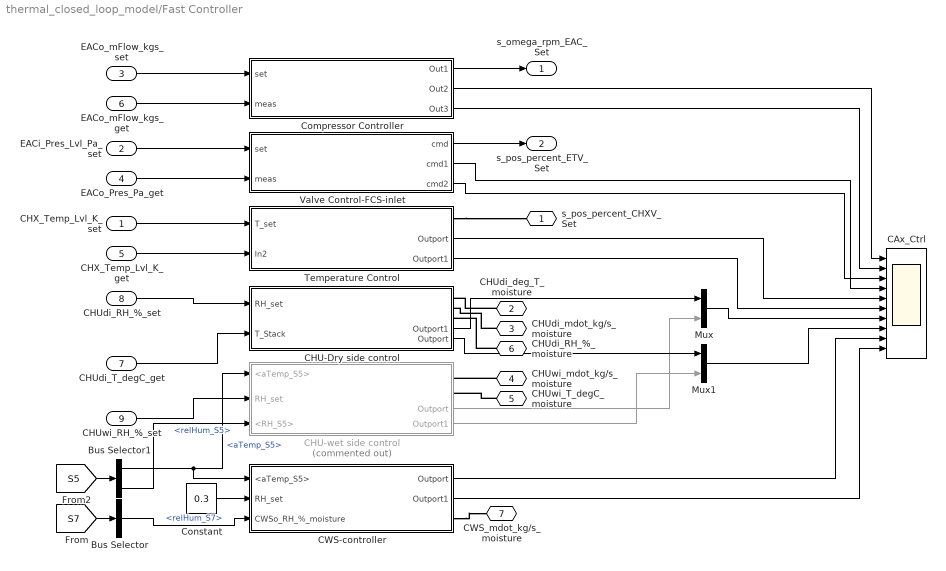
== system thermal_closed_loop_model/Fast Controller ==
  CHX_Temp_Lvl_K_set : Inport
  EACi_Pres_Lvl_Pa_set : Inport  Port=2
  EACo_mFlow_kgs_set : Inport  Port=3
  EACo_Pres_Pa_get : Inport  Port=4
  CHX_Temp_Lvl_K_get : Inport  Port=5
  EACo_mFlow_kgs_get : Inport  Port=6
  CHUdi_T_degC_get : Inport  Port=7
  CHUdi_RH_%_set : Inport  Port=8
  CHUwi_RH_%_set : Inport  Port=9
  Bus Selector : BusSelector  OutputSignals=relHum_S7
  Bus Selector1 : BusSelector  OutputSignals=aTemp_S5,relHum_S5
  CAx_Ctrl : Scope  NumInputPorts=10
  CHU-Dry side control : Subsystem
      settings: PortSchema="{\"entries\":[{\"content\":{\"sides\":[{\"content\":{\"connectorIds\":[\"In1\",\"In2\"]},\"type\":\"ConnectorPlacement.EquallySpacedRectSide\",\"uuid\":\"e04ad6f8-f772-4509-9e44-7e9617907586\"},{\"content\":{\"connectorIds\":[\"RConn1\",\"RConn2\",\"RConn3\",\"Out1\",\"Out2\"],\"side\":\"RIGHT\"},\"type\":\"ConnectorPlacement.EquallySpacedRectSide\",\"uuid\":\"0d864351-c193-45bf-90b1-984eb87a7782\"},{\"content\":{\"side\":\"TOP\"},\"type\":\"ConnectorPlacement.EquallySpacedRectSide\",\"uuid\":\"4c64baeb-8430-45ec-975f-7b4d4952dc8b\"}]},\"type\":\"ConnectorPlacement.EquallySpacedConnector\",\"uuid\":\"5dd74924-e120-426f-b6cd-4773f3c18ed2\"}],\"packageUris\":[\"http://schema.mathworks.com/mf0/Connector/R2020b\"],\"version\":\"1.0\"}"
  CHU-wet side control : Subsystem  Commented=on
      settings: PortSchema="{\"entries\":[{\"content\":{\"sides\":[{\"content\":{\"connectorIds\":[\"In1\",\"In2\",\"In3\"]},\"type\":\"ConnectorPlacement.EquallySpacedRectSide\",\"uuid\":\"5d784ad6-2694-4818-a8d0-e3f25f29943b\"},{\"content\":{\"connectorIds\":[\"RConn1\",\"RConn2\",\"Out1\",\"Out2\"],\"side\":\"RIGHT\"},\"type\":\"ConnectorPlacement.EquallySpacedRectSide\",\"uuid\":\"0f37eddd-db43-448e-bdba-1f3d3b9c7cf9\"},{\"content\":{\"side\":\"TOP\"},\"type\":\"ConnectorPlacement.EquallySpacedRectSide\",\"uuid\":\"2821bd82-ebdd-4ee5-8462-72507a5a1ef1\"}]},\"type\":\"ConnectorPlacement.EquallySpacedConnector\",\"uuid\":\"01309751-94c6-459a-9af4-24f452a07ce7\"}],\"packageUris\":[\"http://schema.mathworks.com/mf0/Connector/R2020b\"],\"version\":\"1.0\"}"
  CWS-controller : Subsystem
  "Compressor Controller " : Subsystem
  Constant : Constant  Value=0.3
  Mux : Mux  Inputs=2
  Mux1 : Mux  Inputs=2
  Temperature Control : Subsystem
      settings: PortSchema="{\"entries\":[{\"content\":{\"sides\":[{\"content\":{\"connectorIds\":[\"In1\",\"In2\"]},\"type\":\"ConnectorPlacement.EquallySpacedRectSide\",\"uuid\":\"e8458165-2262-49de-87f5-2c7bc958bbf7\"},{\"content\":{\"connectorIds\":[\"RConn1\",\"Out1\",\"Out2\"],\"side\":\"RIGHT\"},\"type\":\"ConnectorPlacement.EquallySpacedRectSide\",\"uuid\":\"42ad841b-551f-4f39-a141-2c874d3391ca\"},{\"content\":{\"side\":\"TOP\"},\"type\":\"ConnectorPlacement.EquallySpacedRectSide\",\"uuid\":\"fd6d4917-3fca-4949-93c2-24e90a6fe24c\"}]},\"type\":\"ConnectorPlacement.EquallySpacedConnector\",\"uuid\":\"b641fb00-fee4-4b18-b8cd-d00bddeb3481\"}],\"packageUris\":[\"http://schema.mathworks.com/mf0/Connector/R2020b\"],\"version\":\"1.0\"}"
  Valve Control-FCS-inlet : Subsystem
      settings: PortSchema="{\"entries\":[{\"content\":{\"sides\":[{\"content\":{\"connectorIds\":[\"Out1\",\"Out2\",\"Out3\"]},\"type\":\"ConnectorPlacement.EquallySpacedRectSide\",\"uuid\":\"8b9549d8-0479-4d9d-bb86-2520a85bd308\"},{\"content\":{\"connectorIds\":[\"In1\",\"In2\"],\"side\":\"RIGHT\"},\"type\":\"ConnectorPlacement.EquallySpacedRectSide\",\"uuid\":\"e3096e7f-7009-48fd-960b-05aa908ba84d\"},{\"content\":{\"side\":\"TOP\"},\"type\":\"ConnectorPlacement.EquallySpacedRectSide\",\"uuid\":\"4c3fd166-a148-4bd3-b47b-60debcc19f33\"}]},\"type\":\"ConnectorPlacement.EquallySpacedConnector\",\"uuid\":\"0022fa2c-fa81-4715-9695-0e1425952078\"}],\"packageUris\":[\"http://schema.mathworks.com/mf0/Connector/R2020b\"],\"version\":\"1.0\"}"
  s_pos_percent_CHXV_Set : PMIOPort  Side=Left
  CHUdi_deg_T_moisture : PMIOPort  Port=2  Side=Left
  CHUdi_mdot_kg/s_moisture : PMIOPort  Port=3  Side=Left
  CHUwi_mdot_kg/s_moisture : PMIOPort  Port=4  Side=Left
  CHUwi_T_degC_moisture : PMIOPort  Port=5  Side=Left
  CHUdi_RH_%_moisture : PMIOPort  Port=6  Side=Left
  CWS_mdot_kg/s_moisture : PMIOPort  Port=7  Side=Left
  s_omega_rpm_EAC_Set : Outport
  s_pos_percent_ETV_Set : Outport  Port=2
  wires:
  "Compressor Controller "/1(Out1) -> s_omega_rpm_EAC_Set/1
  CHX_Temp_Lvl_K_get/1 -> Temperature Control/2(In2)
  CHX_Temp_Lvl_K_set/1 -> Temperature Control/1(T_set)
  Valve Control-FCS-inlet/1(cmd) -> s_pos_percent_ETV_Set/1
  EACo_mFlow_kgs_get/1 -> "Compressor Controller "/2(meas)
  EACo_mFlow_kgs_set/1 -> "Compressor Controller "/1(set)
  EACi_Pres_Lvl_Pa_set/1 -> Valve Control-FCS-inlet/1(set)
  EACo_Pres_Pa_get/1 -> Valve Control-FCS-inlet/2(meas)
  "Compressor Controller "/2(Out2) -> CAx_Ctrl/1
  "Compressor Controller "/3(Out3) -> CAx_Ctrl/2
  Valve Control-FCS-inlet/2(cmd1) -> CAx_Ctrl/4
  Valve Control-FCS-inlet/3(cmd2) -> CAx_Ctrl/3
  CHUdi_T_degC_get/1 -> CHU-Dry side control/2(T_Stack)
  CHUdi_RH_%_set/1 -> CHU-Dry side control/1(RH_set)
  CHUwi_RH_%_set/1 -> CHU-wet side control/2(RH_set)
  Bus Selector/1 -> CWS-controller/3(CWSo_RH_%_moisture)  "<relHum_S7>"
  Constant/1 -> CWS-controller/2(RH_set)
  [S7] -> Bus Selector/1
  [S5] -> Bus Selector1/1
  Bus Selector1/1 -> CWS-controller/1(<aTemp_S5>), CHU-wet side control/1(<aTemp_S5>)  "<aTemp_S5>"
  Temperature Control/1(Outport) -> CAx_Ctrl/5
  Temperature Control/2(Outport1) -> CAx_Ctrl/6
  CHU-Dry side control/1(Outport1) -> Mux/1
  CHU-wet side control/1(Outport) -> Mux/2
  CHU-Dry side control/2(Outport) -> Mux1/1
  CHU-wet side control/2(Outport1) -> Mux1/2
  Mux/1 -> CAx_Ctrl/7
  Mux1/1 -> CAx_Ctrl/8
  CWS-controller/1(Outport) -> CAx_Ctrl/9
  CWS-controller/2(Outport1) -> CAx_Ctrl/10
  Bus Selector1/2 -> CHU-wet side control/3(<RH_S5>)  "<relHum_S5>"
  connections:
  Temperature Control/RConn1 -- s_pos_percent_CHXV_Set/RConn1
  CHUdi_deg_T_moisture/RConn1 -- CHU-Dry side control/RConn1
  CHUdi_mdot_kg/s_moisture/RConn1 -- CHU-Dry side control/RConn2
  CHUdi_RH_%_moisture/RConn1 -- CHU-Dry side control/RConn3
  CHUwi_mdot_kg/s_moisture/RConn1 -- CHU-wet side control/RConn1
  CHUwi_T_degC_moisture/RConn1 -- CHU-wet side control/RConn2
  CWS-controller/RConn1 -- CWS_mdot_kg/s_moisture/RConn1

== system thermal_closed_loop_model/Load Cycle(s) ==
  note: TODO: As variant subsystem?
  I_Stack__TB -  Power Cycle : Subsystem  Tag=STV Subsys  LoadFcn=sigbuilder_block('load');  StartFcn=sigbuilder_block('start');  StopFcn=sigbuilder_block('stop');  ClipboardFcn=sigbuilder_block('clipboard');  mask(Sigbuilder block){tuvar=[0:10]}
      mask help: Simulink:masks:SigbuilderBlock_MD
      mask init:
      | if ~strcmp(get_param(bdroot(gcbh),'SimulationStatus'),'stopped') tuvar = sigbuilder_block('maskInit'); end
      settings: CopyFcn=sigbuilder_block('copy');  DeleteFcn=sigbuilder_block('delete');  ModelCloseFcn=sigbuilder_block('modelClose');  PreSaveFcn=sigbuilder_block('preSave');  PauseFcn=sigbuilder_block('pause');  ContinueFcn=sigbuilder_block('continue');  NameChangeFcn=sigbuilder_block('namechange');  OpenFcn=sigbuilder_block('open',[150.6 139.8 551.4 322.2 ]);  CloseFcn=sigbuilder_block('close');
      mask Display: plot(0, 0, 100, 100,[2, 2, 32, 32, 2], [68, 8, 8, 68, 68],[32, 2], [38, 38], [32, 19, 2],[53, 60, 44], [32, 17, 17, 2],[16, 16, 31, 31]);txt = getActiveGroup(gcbh);text(2, 100, txt,'verticalAlignment', 'top');
  P_Stack__MP - Power Demand : Subsystem  Tag=STV Subsys  Commented=on  LoadFcn=sigbuilder_block('load');  StartFcn=sigbuilder_block('start');  StopFcn=sigbuilder_block('stop');  ClipboardFcn=sigbuilder_block('clipboard');  mask(Sigbuilder block){tuvar=[0:10]}
      mask help: Simulink:masks:SigbuilderBlock_MD
      mask init:
      | if ~strcmp(get_param(bdroot(gcbh),'SimulationStatus'),'stopped') tuvar = sigbuilder_block('maskInit'); end
      settings: CopyFcn=sigbuilder_block('copy');  DeleteFcn=sigbuilder_block('delete');  ModelCloseFcn=sigbuilder_block('modelClose');  PreSaveFcn=sigbuilder_block('preSave');  PauseFcn=sigbuilder_block('pause');  ContinueFcn=sigbuilder_block('continue');  NameChangeFcn=sigbuilder_block('namechange');  OpenFcn=sigbuilder_block('open',[5.4 5.4 1141.2 580.8 ]);  CloseFcn=sigbuilder_block('close');
      mask Display: plot(0, 0, 100, 100,[2, 2, 32, 32, 2], [68, 8, 8, 68, 68],[32, 2], [38, 38], [32, 19, 2],[53, 60, 44], [32, 17, 17, 2],[16, 16, 31, 31]);txt = getActiveGroup(gcbh);text(2, 100, txt,'verticalAlignment', 'top');
  Power2Current : Subsystem  Commented=on
  Terminator : Terminator  Commented=on
  I_Stack_A : Outport
  wires:
  P_Stack__MP - Power Demand/1(Stairway) -> Power2Current/1(P_Stack)
  Power2Current/2(V_Stack) -> Terminator/1
  I_Stack__TB -  Power Cycle/1(Stairway) -> I_Stack_A/1

== system thermal_closed_loop_model/MAX-integration_profile ==
  Demux : Demux  Tag=STV Demux  Outputs=1
      settings: DisplayOption=none
  FromWs : FromWorkspace  Tag=STV FromWs  VariableName=tuvar
      SigBuilderData=|
      | common.afterFinalStr = 'Extrapolate'
      | common.sampleTime = 0
      | dataSet.timeRange = [1 1000]
      | dataSet.name = 'Sheet2'
      | sbobj.Groups.Name = 'Sheet2'
      | sbobj.Groups.Signals.Name = 'I'
      | sbobj.Groups.Signals.XData = [1 200 220 400 420 600 620 800 820 1000]
      | sbobj.Groups.Signals.YData = [50 50 200 200 420 420 500 500 600 600]
      | sbobj.Groups.TimeRange = [1 16000]
  I : Outport  Tag=STV Outport
  wires:
  Demux/1 -> I/1
  FromWs/1 -> Demux/1

== system thermal_closed_loop_model/Monitoring ==
  Thermal_Measurement_Bus : Inport
  Controller_Setpoints : Inport  Port=2
  Peripherals_Measurement_Bus : Inport  Port=3
  Add : Sum
  Bus Selector : BusSelector  OutputSignals=Stack Inlet Temperature Setpoint (°C),STCL_dT_SP_degC
  Bus Selector1 : BusSelector  OutputSignals=AuxTCP Rotational Speed Command (rpm),AuxTCP Rotational Speed (rpm)
  Bus Selector2 : BusSelector  OutputSignals="Stack Current: I_A_StN (A),Stack Inlet Temperature: TSens_CLSti 6812 (°C),Stack Outlet Temperature: TSens_CLSto 6820 (°C),TCV Inlet Temperature: TSens_TCVi 6801 (°C),TCV Opening Command (%),TCV Opening  (%),TCP Rotational Speed Command (rpm),TCP Rotational Speed (rpm),TCP Inlet Pressure: pSens_TCPi 6811 (Bar),Stack Inlet Pressure: pSens_CLSti 6812 (Bar),TCV Inlet Pressure: pSens_TCVi 6801 (Bar),Overall Coolant Massflow (kg/s),Hot Circuit Coolant Massflow (kg/s),Cold Circuit Coolant Massflow (kg/s)"
  Main Simulation Results : Scope  NumInputPorts=6
  Mux : Mux  Inputs=3
  Mux1 : Mux  Inputs=3
  Mux2 : Mux  Inputs=2
  Mux3 : Mux
  Mux4 : Mux  Inputs=6
  To Workspace : ToWorkspace  VariableName=simout  SaveFormat=Timeseries  SampleTime=-1
  wires:
  Mux4/1 -> Main Simulation Results/4
  Bus Selector2/9 -> Mux/3  "<TCP Inlet Pressure: pSens_TCPi 6811 (Bar)>"
  Mux3/1 -> Main Simulation Results/3
  Bus Selector2/7 -> Mux3/1  "<TCP Rotational Speed Command (rpm)>"
  Bus Selector2/3 -> Mux4/2  "<Stack Outlet Temperature: TSens_CLSto 6820 (°C)>"
  Mux2/1 -> Main Simulation Results/2
  Thermal_Measurement_Bus/1 -> To Workspace/1, Bus Selector2/1
  Bus Selector2/2 -> Mux4/3, Add/1  "<Stack Inlet Temperature: TSens_CLSti 6812 (°C)>"
  Bus Selector2/6 -> Mux2/2  "<TCV Opening  (%)>"
  Mux/1 -> Main Simulation Results/5
  Bus Selector2/13 -> Mux1/2  "<Hot Circuit Coolant Massflow (kg/s)>"
  Bus Selector2/11 -> Mux/1  "<TCV Inlet Pressure: pSens_TCVi 6801 (Bar)>"
  Bus Selector2/12 -> Mux1/3  "<Overall Coolant Massflow (kg/s)>"
  Mux1/1 -> Main Simulation Results/6
  Bus Selector2/8 -> Mux3/2  "<TCP Rotational Speed (rpm)>"
  Bus Selector2/5 -> Mux2/1  "<TCV Opening Command (%)>"
  Bus Selector2/14 -> Mux1/1  "<Cold Circuit Coolant Massflow (kg/s)>"
  Bus Selector2/10 -> Mux/2  "<Stack Inlet Pressure: pSens_CLSti 6812 (Bar)>"
  Bus Selector2/4 -> Mux4/1  "<TCV Inlet Temperature: TSens_TCVi 6801 (°C)>"
  Bus Selector2/1 -> Main Simulation Results/1  "<Stack Current: I_A_StN (A)>"
  Peripherals_Measurement_Bus/1 -> Bus Selector1/1
  Bus Selector1/1 -> Mux3/3  "<AuxTCP Rotational Speed Command (rpm)>"
  Bus Selector1/2 -> Mux3/4  "<AuxTCP Rotational Speed (rpm)>"
  Bus Selector/1 -> Mux4/6  "<Stack Inlet Temperature Setpoint (°C)>"
  Bus Selector/2 -> Add/2  "<STCL_dT_SP_degC>"
  Add/1 -> Mux4/5  "<Stack Outlet Temperature Setpoint (°C)>"
  [T_TCVi_ref_degC] -> Mux4/4
  Controller_Setpoints/1 -> Bus Selector/1
